simulink model "my_first_model"  (R2019b)
settings: Solver=VariableStepAuto  StartTime=0.0  StopTime=10.0  RelTol=1e-3
values from neighbouring files (symbols this model uses):
  i = ii(p)    [fourfun.m]
settings Model: Creator=Pranshu  LastModifiedBy=Pranshu

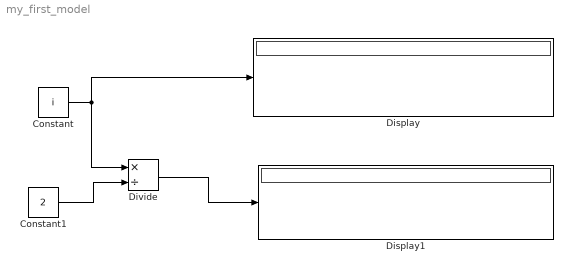
== system my_first_model ==
  Constant : Constant  Value=i
  Constant1 : Constant  Value=2
  Display : Display
  Display1 : Display
  Divide : Product  Inputs=*/
  wires:
  Constant/1 -> Divide/1, Display/1
  Divide/1 -> Display1/1
  Constant1/1 -> Divide/2
